simulink model "AircraftModel_6DoF_SAS"  (R2020b)
settings: Solver=VariableStepAuto  StartTime=0.0  StopTime=20  FixedStep=CNT_StepSize  RelTol=1e-3
values from neighbouring files (symbols this model uses):
  Actuators =     [ControlLaws.mat]    (also in MyTrimReport.mat; TrimState_1_LinearLatModel.mat; TrimState_1_LinearLatModel_Chi.mat; TrimState_1_LinearLatModel_Phasor.mat)
  Aerodynamics =     [ControlLaws.mat]    (also in MyTrimReport.mat; TrimState_1_LinearLatModel.mat; TrimState_1_LinearLatModel_Chi.mat; TrimState_1_LinearLatModel_Phasor.mat)
  CNT_a = 6378137    [AircraftParameters.m]    (also in ControlLaws.mat; MyTrimReport.mat; TrimState_1_LinearLatModel.mat; TrimState_1_LinearLatModel_Chi.mat)
  CNT_f = 0.003352810664747    (= 0.00335281066475)    [AircraftParameters.m]    (also in ControlLaws.mat; MyTrimReport.mat; TrimState_1_LinearLatModel.mat; TrimState_1_LinearLatModel_Chi.mat)
  CNT_g = [0;0;9.81]    [AircraftParameters.m]    (also in ControlLaws.mat = [0 0 9.81]; MyTrimReport.mat = [0 0 9.81]; TrimState_1_LinearLatModel.mat = [0 0 9.81]; TrimState_1_LinearLatModel_Chi.mat = [0 0 9.81])
  CNT_m = 15917    [AircraftParameters.m]    (also in ControlLaws.mat; MyTrimReport.mat; TrimState_1_LinearLatModel.mat; TrimState_1_LinearLatModel_Chi.mat)
  ControlLaws =     [ControlLaws.mat]    (also in MyTrimReport.mat; TrimState_1_LinearLatModel.mat; TrimState_1_LinearLatModel_Chi.mat; TrimState_1_LinearLatModel_Phasor.mat)
  Ixx = 105390    [AircraftParameters.m]    (also in ControlLaws.mat; MyTrimReport.mat; TrimState_1_LinearLatModel.mat; TrimState_1_LinearLatModel_Chi.mat)
  Ixz = 15539    [AircraftParameters.m]    (also in ControlLaws.mat; MyTrimReport.mat; TrimState_1_LinearLatModel.mat; TrimState_1_LinearLatModel_Chi.mat)
  Iyy = 280790    [AircraftParameters.m]    (also in ControlLaws.mat; MyTrimReport.mat; TrimState_1_LinearLatModel.mat; TrimState_1_LinearLatModel_Chi.mat)
  Izz = 350200    [AircraftParameters.m]    (also in ControlLaws.mat; MyTrimReport.mat; TrimState_1_LinearLatModel.mat; TrimState_1_LinearLatModel_Chi.mat)
  Propulsion =     [ControlLaws.mat]    (also in MyTrimReport.mat; TrimState_1_LinearLatModel.mat; TrimState_1_LinearLatModel_Chi.mat; TrimState_1_LinearLatModel_Phasor.mat)
  TrimPoint =     [ControlLaws.mat]    (also in MyTrimReport.mat; TrimState_1_LinearLatModel.mat; TrimState_1_LinearLatModel_Chi.mat; TrimState_1_LinearLatModel_Phasor.mat)
undefined symbols (not defined in the file or in its folder): ampl_p_cmd, beta_cmd, omega_p_cmd, TestSequence
libraries: simulink x32, vrlib x4
(part 1 of 2)
settings Model: Creator=NicolasS  LastModifiedBy=vlsag

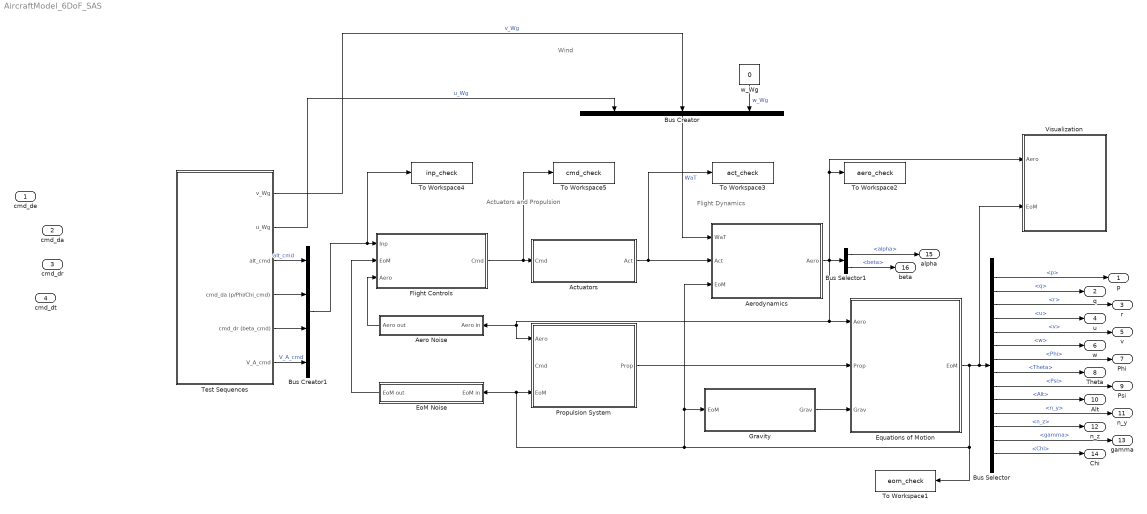
== system AircraftModel_6DoF_SAS ==
  note: Wind
  note: Actuators and Propulsion
  note: Flight Dynamics
  cmd_de : Inport
  cmd_da : Inport  Port=2
  cmd_dr : Inport  Port=3
  cmd_dt : Inport  Port=4
  Actuators : Subsystem
  Aero Noise : Subsystem
  Aerodynamics : Subsystem
  Bus Creator : BusCreator  Inputs=3
  Bus Creator1 : BusCreator  Inputs=4
  Bus Selector : BusSelector  OutputSignals=OOmega_f.p,OOmega_f.q,OOmega_f.r,vv_f.u,vv_f.v,vv_f.w,PPhi.Phi,PPhi.Theta,PPhi.Psi,Position.Alt,nn_f.n_y,nn_f.n_z,TrackData.gamma,TrackData.Chi
  Bus Selector1 : BusSelector  OutputSignals=AirData.alpha,AirData.beta
  EoM Noise : Subsystem
  Equations of Motion : Subsystem
  Flight Controls : Subsystem
  Gravity : Subsystem
  "Propulsion System " : Subsystem
  Test Sequences : Subsystem  InitFcn=|  StopFcn="clear beta_cmd  ampl_p_cmd omega_p_cmd tstart_p_cmd tstart_p_cmd TurnCompensation"
      | if not(exist('TestSequence','var'))
      | TestSequence = 7;
      | end
      | 
      | if not(exist('beta_cmd','var'))
      | beta_cmd = 0;
      | end
      | 
      | if not(exist('ampl_p_cmd','var'))
      | ampl_p_cmd = 0;
      | end
      | 
      | if not(exist('omega_p_cmd','var'))
      | omega_p_cmd = 0;
      | end
      | 
      | if not(exist('tstart_p_cmd','var'))
      | tstart_p_cmd = 0;
      | end
      | 
      | if not(exist('TurnCompensation','var'))
      |  if TestSequence == 4
      |     TurnCompensation = 0;
      |  else
      |     TurnCompensation = 1;
      |  end
      | end
  To Workspace1 : ToWorkspace  VariableName=eom_check  SaveFormat=Timeseries  SampleTime=-1
      settings: Decimation=2
  To Workspace2 : ToWorkspace  VariableName=aero_check  SaveFormat=Timeseries  SampleTime=-1
      settings: Decimation=2
  To Workspace3 : ToWorkspace  VariableName=act_check  SaveFormat=Timeseries  SampleTime=-1
      settings: Decimation=2
  To Workspace4 : ToWorkspace  VariableName=inp_check  SaveFormat=Timeseries  SampleTime=-1
      settings: Decimation=2
  To Workspace5 : ToWorkspace  VariableName=cmd_check  SaveFormat=Timeseries  SampleTime=-1
      settings: Decimation=2
  Visualization : Subsystem
  w_Wg : Constant  Value=0  SampleTime=-1
  p : Outport  Unit=rad/s
  q : Outport  Port=2  Unit=rad/s
  r : Outport  Port=3  Unit=rad/s
  u : Outport  Port=4  Unit=m/s
  v : Outport  Port=5  Unit=m/s
  w : Outport  Port=6  Unit=m/s
  Phi : Outport  Port=7  Unit=rad
  Theta : Outport  Port=8  Unit=rad
  Psi : Outport  Port=9  Unit=rad
  Alt : Outport  Port=10  Unit=m
  n_y : Outport  Port=11
  n_z : Outport  Port=12
  gamma : Outport  Port=13  Unit=rad
  Chi : Outport  Port=14  Unit=rad
  alpha : Outport  Port=15
  beta : Outport  Port=16
  wires:
  Test Sequences/2(u_Wg) -> Bus Creator/1  "u_Wg"
  Actuators/1(Act) -> To Workspace3/1, Aerodynamics/2(Act)
  Aerodynamics/1(Aero) -> To Workspace2/1, Visualization/1(Aero), Bus Selector1/1, Equations of Motion/1(Aero), Aero Noise/1(Aero in), "Propulsion System "/1(Aero)
  w_Wg/1 -> Bus Creator/3  "w_Wg"
  Equations of Motion/1(EoM) -> To Workspace1/1, Aerodynamics/3(EoM), Gravity/1(EoM), EoM Noise/1(EoM in), "Propulsion System "/3(EoM), Visualization/2(EoM), Bus Selector/1
  "Propulsion System "/1(Prop) -> Equations of Motion/2(Prop)
  Gravity/1(Grav) -> Equations of Motion/3(Grav)
  Bus Creator/1 -> Aerodynamics/1(WaT)  "WaT"
  Bus Selector1/2 -> beta/1  "<beta>"
  Test Sequences/1(v_Wg) -> Bus Creator/2  "v_Wg"
  Bus Selector/3 -> r/1  "<r>"
  Bus Selector/9 -> Psi/1  "<Psi>"
  Bus Selector/7 -> Phi/1  "<Phi>"
  Bus Selector/1 -> p/1  "<p>"
  Bus Selector/11 -> n_y/1  "<n_y>"
  Bus Selector1/1 -> alpha/1  "<alpha>"
  Bus Selector/2 -> q/1  "<q>"
  Bus Selector/6 -> w/1  "<w>"
  Bus Selector/4 -> u/1  "<u>"
  Bus Selector/12 -> n_z/1  "<n_z>"
  Bus Selector/10 -> Alt/1  "<Alt>"
  Bus Selector/8 -> Theta/1  "<Theta>"
  Bus Selector/13 -> gamma/1  "<gamma>"
  Bus Selector/14 -> Chi/1  "<Chi>"
  Bus Selector/5 -> v/1  "<v>"
  Flight Controls/1(Cmd) -> To Workspace5/1, Actuators/1(Cmd)
  Aero Noise/1(Aero out) -> Flight Controls/3(Aero)
  EoM Noise/1(EoM out) -> Flight Controls/2(EoM)
  Bus Creator1/1 -> To Workspace4/1, Flight Controls/1(Inp)
  Test Sequences/4(cmd_da (p/Phi/Chi_cmd)) -> Bus Creator1/2
  Test Sequences/3(alt_cmd) -> Bus Creator1/1  "alt_cmd"
  Test Sequences/5(cmd_dr (beta_cmd)) -> Bus Creator1/3
  Test Sequences/6(V_A_cmd) -> Bus Creator1/4  "V_A_cmd"

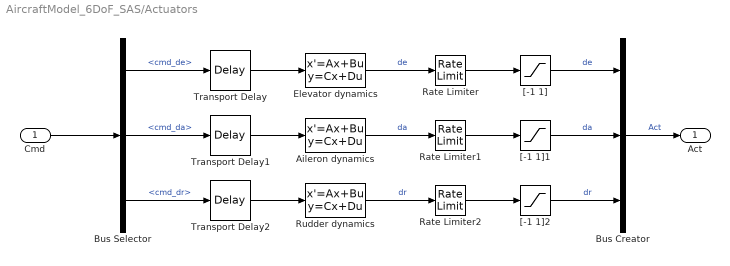
== system AircraftModel_6DoF_SAS/Actuators ==
  Cmd : Inport  OutDataTypeStr=Bus: Cmd
  Aileron dynamics : StateSpace  A=Actuators.Act_a.A  B=Actuators.Act_a.B  C=Actuators.Act_a.C  D=Actuators.Act_a.D  InitialCondition=TrimPoint.States.dabar  ContinuousStateAttributes='da'
  Bus Creator : BusCreator  Inputs=3  OutDataTypeStr=Bus: Act
  Bus Selector : BusSelector  OutputSignals=cmd_de,cmd_da,cmd_dr
  Elevator dynamics : StateSpace  A=Actuators.Act_e.A  B=Actuators.Act_e.B  C=Actuators.Act_e.C  D=Actuators.Act_e.D  InitialCondition=TrimPoint.States.debar  ContinuousStateAttributes='de'
  Rate Limiter : RateLimiter  RisingSlewLimit=max(Actuators.RateLimits.udot_max_He)  FallingSlewLimit=min(Actuators.RateLimits.udot_max_He)  SampleTimeMode=inherited
  Rate Limiter1 : RateLimiter  RisingSlewLimit=max(Actuators.RateLimits.udot_max_Ha)  FallingSlewLimit=min(Actuators.RateLimits.udot_max_Ha)  SampleTimeMode=inherited
  Rate Limiter2 : RateLimiter  RisingSlewLimit=max(Actuators.RateLimits.udot_max_Hr)  FallingSlewLimit=min(Actuators.RateLimits.udot_max_Hr)  SampleTimeMode=inherited
  Rudder dynamics : StateSpace  A=Actuators.Act_r.A  B=Actuators.Act_r.B  C=Actuators.Act_r.C  D=Actuators.Act_r.D  InitialCondition=TrimPoint.States.drbar  ContinuousStateAttributes='dr'
  Transport Delay : TransportDelay  DelayTime=Actuators.Delays.tau_de  InitialOutput=TrimPoint.States.debar  TransDelayFeedthrough=on
  Transport Delay1 : TransportDelay  DelayTime=Actuators.Delays.tau_da  InitialOutput=TrimPoint.States.dabar  TransDelayFeedthrough=on
  Transport Delay2 : TransportDelay  DelayTime=Actuators.Delays.tau_dr  InitialOutput=TrimPoint.States.drbar  TransDelayFeedthrough=on
  "[-1 1]" : Saturate  UpperLimit=max(Actuators.Limits.u_max_He)  LowerLimit=min(Actuators.Limits.u_max_He)
  "[-1 1]1" : Saturate  UpperLimit=max(Actuators.Limits.u_max_Ha)  LowerLimit=min(Actuators.Limits.u_max_Ha)
  "[-1 1]2" : Saturate  UpperLimit=max(Actuators.Limits.u_max_Hr)  LowerLimit=min(Actuators.Limits.u_max_Hr)
  Act : Outport  OutDataTypeStr=Bus: Act
  wires:
  Elevator dynamics/1 -> Rate Limiter/1  "de"
  "[-1 1]1"/1 -> Bus Creator/2  "da"
  Rudder dynamics/1 -> Rate Limiter2/1  "dr"
  Transport Delay1/1 -> Aileron dynamics/1
  Cmd/1 -> Bus Selector/1
  "[-1 1]"/1 -> Bus Creator/1  "de"
  Bus Selector/1 -> Transport Delay/1  "<cmd_de>"
  Transport Delay/1 -> Elevator dynamics/1
  "[-1 1]2"/1 -> Bus Creator/3  "dr"
  Transport Delay2/1 -> Rudder dynamics/1
  Aileron dynamics/1 -> Rate Limiter1/1  "da"
  Bus Selector/3 -> Transport Delay2/1  "<cmd_dr>"
  Bus Creator/1 -> Act/1  "Act"
  Bus Selector/2 -> Transport Delay1/1  "<cmd_da>"
  Rate Limiter/1 -> "[-1 1]"/1
  Rate Limiter1/1 -> "[-1 1]1"/1
  Rate Limiter2/1 -> "[-1 1]2"/1

== system AircraftModel_6DoF_SAS/Aero Noise ==
  Aero in : Inport  OutDataTypeStr=Bus: Aero
  Band-Limited White Noise1 : simulink/Sources/Band-Limited White Noise  Cov=1E-7  Ts=0.01  seed=5749
  Band-Limited White Noise8 : simulink/Sources/Band-Limited White Noise  Cov=1E-7  Ts=0.01  seed=3324
  Band-Limited White Noise9 : simulink/Sources/Band-Limited White Noise  Cov=1E-3  Ts=0.05  seed=8153
  Bus Creator2 : BusCreator  Inputs=7  OutDataTypeStr=Bus: Aero
  Bus Creator3 : BusCreator  Inputs=7  OutDataTypeStr=Bus: AirData
  Bus Selector : BusSelector  OutputSignals=AirData.u_Af,AirData.v_Af,AirData.w_Af,AirData.V_A,AirData.p_dyn,AirData.alpha,AirData.beta,X_A,Y_A,Z_A,L_A,M_A,N_A
  Sum1 : Sum  Inputs=++|
  Sum2 : Sum  Inputs=++|
  Sum3 : Sum  Inputs=++|
  Aero out : Outport  OutDataTypeStr=Bus: Aero
  wires:
  Aero in/1 -> Bus Selector/1
  Bus Creator3/1 -> Bus Creator2/1  "AirData"
  Bus Selector/7 -> Sum2/2  "<beta>"
  Bus Selector/8 -> Bus Creator2/2  "<X_A>"
  Bus Creator2/1 -> Aero out/1  "Aero"
  Bus Selector/1 -> Bus Creator3/1  "<u_Af>"
  Bus Selector/3 -> Bus Creator3/3  "<w_Af>"
  Bus Selector/4 -> Sum3/2  "<V_A>"
  Bus Selector/6 -> Sum1/2  "<alpha>"
  Band-Limited White Noise8/1 -> Sum1/1
  Sum1/1 -> Bus Creator3/6  "alpha"
  Bus Selector/5 -> Bus Creator3/5  "<p_dyn>"
  Band-Limited White Noise9/1 -> Sum3/1
  Sum3/1 -> Bus Creator3/4  "V_A"
  Bus Selector/2 -> Bus Creator3/2  "<v_Af>"
  Bus Selector/9 -> Bus Creator2/3  "<Y_A>"
  Bus Selector/10 -> Bus Creator2/4  "<Z_A>"
  Bus Selector/11 -> Bus Creator2/5  "<L_A>"
  Bus Selector/12 -> Bus Creator2/6  "<M_A>"
  Bus Selector/13 -> Bus Creator2/7  "<N_A>"
  Band-Limited White Noise1/1 -> Sum2/1
  Sum2/1 -> Bus Creator3/7  "beta"

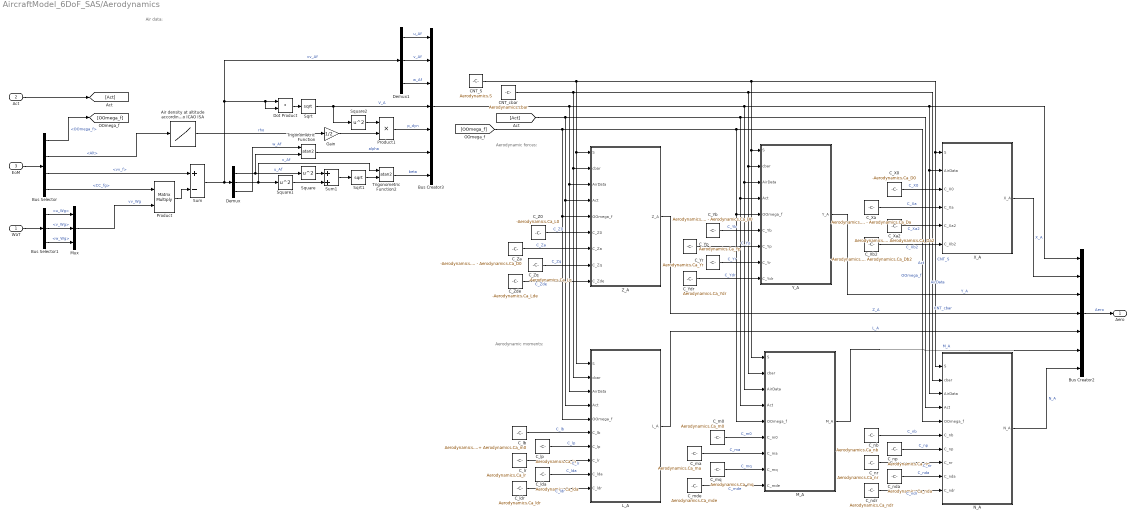
== system AircraftModel_6DoF_SAS/Aerodynamics ==
  note: Air data:
  note: Aerodynamic moments:
  note: Aerodynamic forces:
  WaT : Inport  OutDataTypeStr=Bus: WaT
  Act : Inport  Port=2  OutDataTypeStr=Bus: Act
  EoM : Inport  Port=3  OutDataTypeStr=Bus: EoM
  Air density at altitude according to ICAO ISA : Lookup_n-D  NumberOfTableDimensions=1  BreakpointsForDimension1=Aerodynamics.LUT_Alt  Table=Aerodynamics.LUT_rho  ExtrapMethod=Clip  InternalRulePriority=Speed  RndMeth=Simplest  InputSameDT=on
  Bus Creator2 : BusCreator  Inputs=7  OutDataTypeStr=Bus: Aero
  Bus Creator3 : BusCreator  Inputs=7  OutDataTypeStr=Bus: AirData
  Bus Selector : BusSelector  OutputSignals=OOmega_f,Position.Alt,vv_f,CC.CC_fg
  Bus Selector1 : BusSelector  OutputSignals=u_Wg,v_Wg,w_Wg
  CNT_S : Constant  Value=Aerodynamics.S  OutDataTypeStr=double  SampleTime=-1
  CNT_cbar : Constant  Value=Aerodynamics.cbar  OutDataTypeStr=double  SampleTime=-1
  C_X0 : Constant  Value=-Aerodynamics.Ca_D0  VectorParams1D=off  OutDataTypeStr=double  SampleTime=-1
  C_Xa : Constant  Value=Aerodynamics.Ca_L0 - Aerodynamics.Ca_Da  VectorParams1D=off  OutDataTypeStr=double  SampleTime=-1
  C_Xa2 : Constant  Value=Aerodynamics.Ca_La - Aerodynamics.Ca_Da2  VectorParams1D=off  OutDataTypeStr=double  SampleTime=-1
  C_Xb2 : Constant  Value=-Aerodynamics.Ca_Yb - Aerodynamics.Ca_Db2  VectorParams1D=off  OutDataTypeStr=double  SampleTime=-1
  C_Yb : Constant  Value=Aerodynamics.Ca_Yb - Aerodynamics.Ca_D0  VectorParams1D=off  OutDataTypeStr=double  SampleTime=-1
  C_Ydr : Constant  Value=Aerodynamics.Ca_Ydr  VectorParams1D=off  OutDataTypeStr=double  SampleTime=-1
  C_Yp : Constant  Value=Aerodynamics.Ca_Yp  VectorParams1D=off  OutDataTypeStr=double  SampleTime=-1
  C_Yr : Constant  Value=Aerodynamics.Ca_Yr  VectorParams1D=off  OutDataTypeStr=double  SampleTime=-1
  C_Z0 : Constant  Value=-Aerodynamics.Ca_L0  VectorParams1D=off  OutDataTypeStr=double  SampleTime=-1
  C_Za : Constant  Value=-Aerodynamics.Ca_La - Aerodynamics.Ca_D0  VectorParams1D=off  OutDataTypeStr=double  SampleTime=-1
  C_Zde : Constant  Value=-Aerodynamics.Ca_Lde  VectorParams1D=off  OutDataTypeStr=double  SampleTime=-1
  C_Zq : Constant  Value=-Aerodynamics.Ca_Lq  VectorParams1D=off  OutDataTypeStr=double  SampleTime=-1
  C_lb : Constant  Value=Aerodynamics.Ca_lb + Aerodynamics.Ca_m0  VectorParams1D=off  OutDataTypeStr=double  SampleTime=-1
  C_lda : Constant  Value=Aerodynamics.Ca_lda  VectorParams1D=off  OutDataTypeStr=double  SampleTime=-1
  C_ldr : Constant  Value=Aerodynamics.Ca_ldr  VectorParams1D=off  OutDataTypeStr=double  SampleTime=-1
  C_lp : Constant  Value=Aerodynamics.Ca_lp  VectorParams1D=off  OutDataTypeStr=double  SampleTime=-1
  C_lr : Constant  Value=Aerodynamics.Ca_lr  VectorParams1D=off  OutDataTypeStr=double  SampleTime=-1
  C_m0 : Constant  Value=Aerodynamics.Ca_m0  VectorParams1D=off  OutDataTypeStr=double  SampleTime=-1
  C_ma : Constant  Value=Aerodynamics.Ca_ma  VectorParams1D=off  OutDataTypeStr=double  SampleTime=-1
  C_mde : Constant  Value=Aerodynamics.Ca_mde  VectorParams1D=off  OutDataTypeStr=double  SampleTime=-1
  C_mq : Constant  Value=Aerodynamics.Ca_mq  VectorParams1D=off  OutDataTypeStr=double  SampleTime=-1
  C_nb : Constant  Value=Aerodynamics.Ca_nb  VectorParams1D=off  OutDataTypeStr=double  SampleTime=-1
  C_nda : Constant  Value=Aerodynamics.Ca_nda  VectorParams1D=off  OutDataTypeStr=double  SampleTime=-1
  C_ndr : Constant  Value=Aerodynamics.Ca_ndr  VectorParams1D=off  OutDataTypeStr=double  SampleTime=-1
  C_np : Constant  Value=Aerodynamics.Ca_np  VectorParams1D=off  OutDataTypeStr=double  SampleTime=-1
  C_nr : Constant  Value=Aerodynamics.Ca_nr  VectorParams1D=off  OutDataTypeStr=double  SampleTime=-1
  Demux : Demux  Outputs=3
  Demux1 : Demux  Outputs=3
  Dot Product : DotProduct  InputSameDT=on  OutDataTypeStr=Inherit: Inherit via internal rule
  Gain : Gain  Gain=1/2
  L_A : MATLAB Function  TreatAsAtomicUnit=on
  M_A : MATLAB Function  TreatAsAtomicUnit=on
  Mux : Mux  Inputs=3
  N_A : MATLAB Function  TreatAsAtomicUnit=on
  Product : Product  Multiplication=Matrix(*)
  Product1 : Product
  Sqrt : Sqrt  SaturateOnIntegerOverflow=on
  Sqrt1 : Sqrt  SaturateOnIntegerOverflow=on
  Square : Math  Operator=square  SaturateOnIntegerOverflow=on
  Square1 : Math  Operator=square  SaturateOnIntegerOverflow=on
  Square2 : Math  Operator=square  SaturateOnIntegerOverflow=on
  Sum : Sum  Inputs=+-
  Sum1 : Sum
  Trigonometric Function : Trigonometry  Operator=atan2
  Trigonometric Function2 : Trigonometry  Operator=atan2
  X_A : MATLAB Function  TreatAsAtomicUnit=on
  Y_A : MATLAB Function  TreatAsAtomicUnit=on
  Z_A : MATLAB Function  TreatAsAtomicUnit=on
  Aero : Outport  OutDataTypeStr=Bus: Aero
  wires:
  Demux1/3 -> Bus Creator3/3  "w_Af"
  C_lp/1 -> L_A/7(C_lp)  "C_lp"
  Act/1 -> [Act]
  N_A/1(N_A) -> Bus Creator2/7  "N_A"
  C_nb/1 -> N_A/6(C_nb)  "C_nb"
  C_ldr/1 -> L_A/10(C_ldr)  "C_ldr"
  C_m0/1 -> M_A/6(C_m0)  "C_m0"
  C_Zq/1 -> Z_A/8(C_Zq)  "C_Zq"
  [OOmega_f] -> N_A/5(OOmega_f), M_A/5(OOmega_f), Y_A/5(OOmega_f), L_A/5(OOmega_f), Z_A/5(OOmega_f)  "OOmega_f"
  C_lr/1 -> L_A/8(C_lr)  "C_lr"
  C_mq/1 -> M_A/8(C_mq)  "C_mq"
  Air density at altitude according to ICAO ISA/1 -> Gain/1  "rho"
  C_Z0/1 -> Z_A/6(C_Z0)  "C_Z0"
  Square/1 -> Sum1/1
  X_A/1(X_A) -> Bus Creator2/2  "X_A"
  Trigonometric Function2/1 -> Bus Creator3/7  "beta"
  C_Yr/1 -> Y_A/8(C_Yr)  "C_Yr"
  C_Yb/1 -> Y_A/6(C_Yb)  "C_Yb"
  Demux1/2 -> Bus Creator3/2  "v_Af"
  Dot Product/1 -> Sqrt/1
  C_ma/1 -> M_A/7(C_ma)  "C_ma"
  C_nda/1 -> N_A/9(C_nda)  "C_nda"
  C_Xa/1 -> X_A/4(C_Xa)  "C_Xa"
  C_lb/1 -> L_A/6(C_lb)  "C_lb"
  Sum/1 -> Demux/1, Demux1/1, Dot Product/2, Dot Product/1  "vv_Af"
  C_Xa2/1 -> X_A/5(C_Xa2)  "C_Xa2"
  C_Ydr/1 -> Y_A/9(C_Ydr)  "C_Ydr"
  C_Xb2/1 -> X_A/6(C_Xb2)  "C_Xb2"
  Y_A/1(Y_A) -> Bus Creator2/3  "Y_A"
  C_Za/1 -> Z_A/7(C_Za)  "C_Za"
  CNT_S/1 -> N_A/1(S), X_A/1(S), M_A/1(S), Y_A/1(S), L_A/1(S), Z_A/1(S)  "CNT_S"
  C_nr/1 -> N_A/8(C_nr)  "C_nr"
  Bus Creator2/1 -> Aero/1  "Aero"
  C_mde/1 -> M_A/9(C_mde)  "C_mde"
  [Act] -> N_A/4(Act), M_A/4(Act), Y_A/4(Act), L_A/4(Act), Z_A/4(Act)  "Act"
  Demux/3 -> Trigonometric Function/1  "w_Af"
  C_X0/1 -> X_A/3(C_X0)  "C_X0"
  C_np/1 -> N_A/7(C_np)  "C_np"
  Demux/2 -> Square1/1, Trigonometric Function2/1  "v_Af"
  C_Yp/1 -> Y_A/7(C_Yp)  "C_Yp"
  C_ndr/1 -> N_A/10(C_ndr)  "C_ndr"
  Demux/1 -> Square/1, Trigonometric Function/2  "u_Af"
  Bus Creator3/1 -> L_A/3(AirData), Z_A/3(AirData), Bus Creator2/1, N_A/3(AirData), X_A/2(AirData), M_A/3(AirData), Y_A/3(AirData)  "AirData"
  M_A/1(M_A) -> Bus Creator2/6  "M_A"
  Sqrt1/1 -> Trigonometric Function2/2
  Bus Selector/2 -> Air density at altitude according to ICAO ISA/1  "<Alt>"
  C_Zde/1 -> Z_A/9(C_Zde)  "C_Zde"
  Gain/1 -> Product1/2
  Product/1 -> Sum/2
  C_lda/1 -> L_A/9(C_lda)  "C_lda"
  L_A/1(L_A) -> Bus Creator2/5  "L_A"
  Demux1/1 -> Bus Creator3/1  "u_Af"
  Z_A/1(Z_A) -> Bus Creator2/4  "Z_A"
  Product1/1 -> Bus Creator3/5  "p_dyn"
  Sqrt/1 -> Square2/1, Bus Creator3/4  "V_A"
  CNT_cbar/1 -> N_A/2(cbar), M_A/2(cbar), Y_A/2(cbar), L_A/2(cbar), Z_A/2(cbar)  "CNT_cbar"
  Trigonometric Function/1 -> Bus Creator3/6  "alpha"
  Bus Selector/3 -> Sum/1  "<vv_f>"
  Sum1/1 -> Sqrt1/1
  EoM/1 -> Bus Selector/1
  Bus Selector/1 -> [OOmega_f]  "<OOmega_f>"
  Bus Selector/4 -> Product/1  "<CC_fg>"
  Square2/1 -> Product1/1
  Square1/1 -> Sum1/2
  WaT/1 -> Bus Selector1/1
  Bus Selector1/1 -> Mux/1  "<u_Wg>"
  Bus Selector1/2 -> Mux/2  "<v_Wg>"
  Bus Selector1/3 -> Mux/3  "<w_Wg>"
  Mux/1 -> Product/2  "vv_Wg"

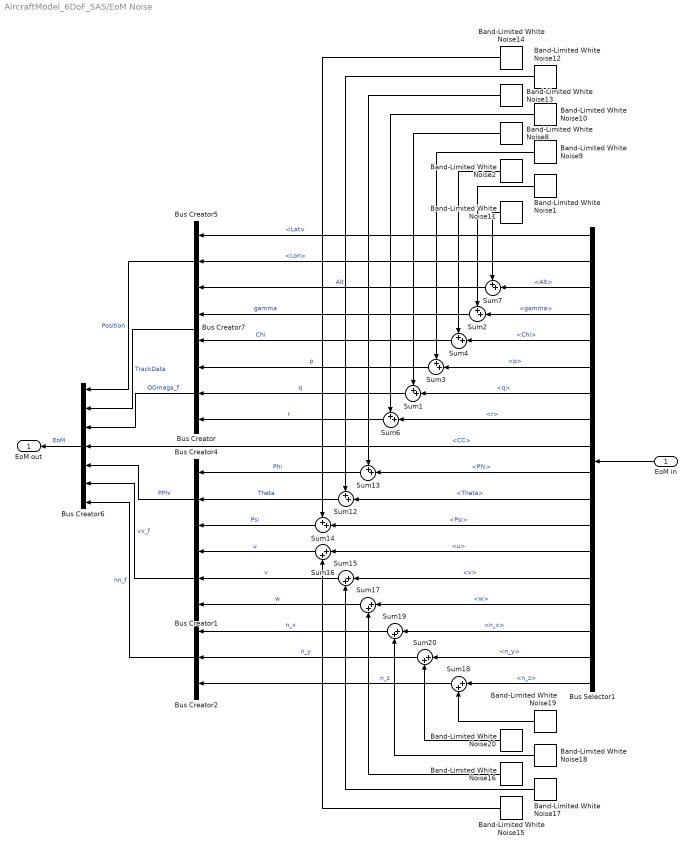
== system AircraftModel_6DoF_SAS/EoM Noise ==
  EoM in : Inport  OutDataTypeStr=Bus: EoM
  Band-Limited White Noise1 : simulink/Sources/Band-Limited White Noise  Cov=1E-7  Ts=0.01  seed=1102
  Band-Limited White Noise10 : simulink/Sources/Band-Limited White Noise  Cov=1E-6  Ts=0.01  seed=66897
  Band-Limited White Noise11 : simulink/Sources/Band-Limited White Noise  Cov=1E-4  Ts=0.1  seed=6874
  Band-Limited White Noise12 : simulink/Sources/Band-Limited White Noise  Cov=5E-7  Ts=0.01  seed=45875
  Band-Limited White Noise13 : simulink/Sources/Band-Limited White Noise  Cov=5E-7  Ts=0.01  seed=74148
  Band-Limited White Noise14 : simulink/Sources/Band-Limited White Noise  Cov=5E-7  Ts=0.01  seed=3514
  Band-Limited White Noise15 : simulink/Sources/Band-Limited White Noise  Cov=5E-5  Ts=0.1  seed=54769
  Band-Limited White Noise16 : simulink/Sources/Band-Limited White Noise  Cov=1E-4  Ts=0.01  seed=6932
  Band-Limited White Noise17 : simulink/Sources/Band-Limited White Noise  Cov=1E-4  Ts=0.01  seed=4485
  Band-Limited White Noise18 : simulink/Sources/Band-Limited White Noise  Cov=1E-5  Ts=0.01  seed=11452
  Band-Limited White Noise19 : simulink/Sources/Band-Limited White Noise  Cov=1E-5  Ts=0.01  seed=3324
  Band-Limited White Noise2 : simulink/Sources/Band-Limited White Noise  Cov=1E-7  Ts=0.1  seed=2201
  Band-Limited White Noise20 : simulink/Sources/Band-Limited White Noise  Cov=1E-5  Ts=0.01  seed=58967
  Band-Limited White Noise8 : simulink/Sources/Band-Limited White Noise  Cov=1E-6  Ts=0.01  seed=[23341]
  Band-Limited White Noise9 : simulink/Sources/Band-Limited White Noise  Cov=1E-6  Ts=0.01  seed=1147
  Bus Creator : BusCreator  Inputs=3  OutDataTypeStr=Bus: OOmega_f
  Bus Creator1 : BusCreator  Inputs=3  OutDataTypeStr=Bus: vv_f
  Bus Creator2 : BusCreator  Inputs=3  OutDataTypeStr=Bus: nn_f
  Bus Creator4 : BusCreator  Inputs=3  OutDataTypeStr=Bus: PPhi
  Bus Creator5 : BusCreator  Inputs=3  OutDataTypeStr=Bus: Position
  Bus Creator6 : BusCreator  Inputs=7  OutDataTypeStr=Bus: EoM
  Bus Creator7 : BusCreator  Inputs=2  OutDataTypeStr=Bus: TrackData
  Bus Selector1 : BusSelector  OutputSignals=Position.Lat,Position.Lon,Position.Alt,TrackData.gamma,TrackData.Chi,OOmega_f.p,OOmega_f.q,OOmega_f.r,CC,PPhi.Phi,PPhi.Theta,PPhi.Psi,vv_f.u,vv_f.v,vv_f.w,nn_f.n_x,nn_f.n_y,nn_f.n_z
  Sum{1..4,6..7,12..14} (9 alike) : Sum  Inputs=++|
  Sum{15..20} (6 alike) : Sum  Inputs=|++
  EoM out : Outport  OutDataTypeStr=Bus: EoM
  wires:
  EoM in/1 -> Bus Selector1/1
  Bus Selector1/6 -> Sum3/2  "<p>"
  Bus Selector1/7 -> Sum1/2  "<q>"
  Band-Limited White Noise9/1 -> Sum3/1
  Bus Selector1/8 -> Sum6/2  "<r>"
  Band-Limited White Noise10/1 -> Sum6/1
  Band-Limited White Noise11/1 -> Sum7/1
  Bus Selector1/3 -> Sum7/2  "<Alt>"
  Band-Limited White Noise12/1 -> Sum12/1
  Bus Selector1/10 -> Sum13/2  "<Phi>"
  Bus Selector1/11 -> Sum12/2  "<Theta>"
  Bus Selector1/12 -> Sum14/2  "<Psi>"
  Band-Limited White Noise13/1 -> Sum13/1
  Band-Limited White Noise14/1 -> Sum14/1
  Bus Selector1/16 -> Sum19/1  "<n_x>"
  Bus Selector1/17 -> Sum20/1  "<n_y>"
  Bus Selector1/18 -> Sum18/1  "<n_z>"
  Bus Selector1/15 -> Sum17/1  "<w>"
  Bus Selector1/13 -> Sum16/1  "<u>"
  Band-Limited White Noise16/1 -> Sum17/2
  Band-Limited White Noise15/1 -> Sum16/2
  Bus Selector1/14 -> Sum15/1  "<v>"
  Band-Limited White Noise17/1 -> Sum15/2
  Band-Limited White Noise19/1 -> Sum18/2
  Band-Limited White Noise18/1 -> Sum19/2
  Band-Limited White Noise20/1 -> Sum20/2
  Bus Selector1/1 -> Bus Creator5/1  "<Lat>"
  Bus Selector1/2 -> Bus Creator5/2  "<Lon>"
  Sum19/1 -> Bus Creator2/1  "n_x"
  Sum20/1 -> Bus Creator2/2  "n_y"
  Sum18/1 -> Bus Creator2/3  "n_z"
  Sum15/1 -> Bus Creator1/2  "v"
  Sum16/1 -> Bus Creator1/1  "u"
  Sum17/1 -> Bus Creator1/3  "w"
  Sum7/1 -> Bus Creator5/3  "Alt"
  Sum6/1 -> Bus Creator/3  "r"
  Sum1/1 -> Bus Creator/2  "q"
  Sum3/1 -> Bus Creator/1  "p"
  Sum13/1 -> Bus Creator4/1  "Phi"
  Bus Selector1/9 -> Bus Creator6/4  "<CC>"
  Sum12/1 -> Bus Creator4/2  "Theta"
  Sum14/1 -> Bus Creator4/3  "Psi"
  Bus Creator5/1 -> Bus Creator6/1  "Position"
  Bus Creator/1 -> Bus Creator6/3  "OOmega_f"
  Bus Creator4/1 -> Bus Creator6/5  "PPhi"
  Bus Creator1/1 -> Bus Creator6/6  "vv_f"
  Bus Creator2/1 -> Bus Creator6/7  "nn_f"
  Bus Creator6/1 -> EoM out/1  "EoM"
  Band-Limited White Noise8/1 -> Sum1/1
  Bus Creator7/1 -> Bus Creator6/2  "TrackData"
  Band-Limited White Noise1/1 -> Sum2/1
  Bus Selector1/5 -> Sum4/2  "<Chi>"
  Band-Limited White Noise2/1 -> Sum4/1
  Bus Selector1/4 -> Sum2/2  "<gamma>"
  Sum2/1 -> Bus Creator7/1  "gamma"
  Sum4/1 -> Bus Creator7/2  "Chi"

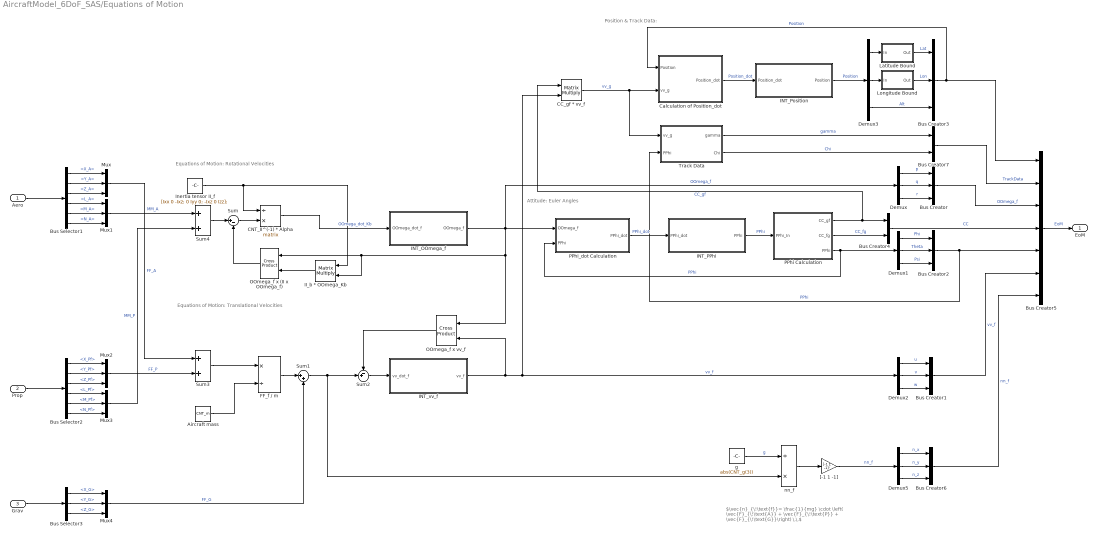
== system AircraftModel_6DoF_SAS/Equations of Motion ==
  note: Equations of Motion: Translational Velocities
  note: Equations of Motion: Rotational Velocities
  note: Attitude: Euler Angles
  note: Position & Track Data:
  note: $\vec{n}_{\!\text{f}}= \frac{1}{mg} \cdot \left( \vec{F}_{\!\text{A}} + \vec{F}_{\!\text{P}} + \vec{F}_{\!\text{G}}\right) \,\,$
  Aero : Inport  OutDataTypeStr=Bus: Aero
  Prop : Inport  Port=2  OutDataTypeStr=Bus: Prop
  Grav : Inport  Port=3  OutDataTypeStr=Bus: Grav
  Aircraft mass : Constant  Value=CNT_m  SampleTime=-1
  Bus Creator : BusCreator  Inputs=3  OutDataTypeStr=Bus: OOmega_f
  Bus Creator1 : BusCreator  Inputs=3  OutDataTypeStr=Bus: vv_f
  Bus Creator2 : BusCreator  Inputs=3  OutDataTypeStr=Bus: PPhi
  Bus Creator3 : BusCreator  Inputs=3  OutDataTypeStr=Bus: Position
  Bus Creator4 : BusCreator  Inputs=2  OutDataTypeStr=Bus: CC
  Bus Creator5 : BusCreator  Inputs=7  OutDataTypeStr=Bus: EoM
  Bus Creator6 : BusCreator  Inputs=3  OutDataTypeStr=Bus: nn_f
  Bus Creator7 : BusCreator  Inputs=2  OutDataTypeStr=Bus: TrackData
  Bus Selector1 : BusSelector  OutputSignals=X_A,Y_A,Z_A,L_A,M_A,N_A
  Bus Selector2 : BusSelector  OutputSignals=X_Pf,Y_Pf,Z_Pf,L_Pf,M_Pf,N_Pf
  Bus Selector3 : BusSelector  OutputSignals=X_G,Y_G,Z_G
  CC_gf * vv_f : Product  Multiplication=Matrix(*)  RndMeth=Zero
  CNT_II^(-1) * Alpha : Product  Inputs=/*  Multiplication=Matrix(*)
  Calculation of Position_dot : Subsystem
  Demux{,1..3,5} (5 alike) : Demux  Outputs=3
  FF_f / m : Product  Inputs=*/
  II_b * OOmega_Kb : Product  Multiplication=Matrix(*)  RndMeth=Zero
  INT_OOmega_f : Subsystem
  INT_PPhi : Subsystem
  INT_Position : Subsystem
  INT_vv_f : Subsystem
  Inertia tensor II_f : Constant  Value=[Ixx 0 -Ixz; 0 Iyy 0; -Ixz 0 Izz];  SampleTime=-1
  Latitude Bound : Subsystem  mask(Latitude bound){}
      mask help: Bounds the latitude to [-pi/2, pi/2]. When the lower bound is exceeded the latitude is increasing again; when the upper bound is exceeded the latitude is decreasing.
  Longitude Bound : Subsystem  mask(Longitude bound){}
      mask help: Bounds the longitude to [-pi, pi]. When -pi bound is exceeded the longitude wraps back to pi; when the pi bound is exceeded the longitude wraps back to -pi.
  Mux{,1..4} (5 alike) : Mux  Inputs=3
  OOmega_f x (II x OOmega_f) : vrlib/Utilities/Cross Product
  OOmega_f x vv_f : vrlib/Utilities/Cross Product
  PPhi Calculation : MATLAB Function  TreatAsAtomicUnit=on
  PPhi_dot Calculation : MATLAB Function  TreatAsAtomicUnit=on
  Sum : Sum  Inputs=|+-
  Sum1 : Sum  Inputs=|++
  Sum2 : Sum  Inputs=-+|
  Sum3 : Sum
  Sum4 : Sum
  Track Data : Subsystem
  "[-1 1 -1]" : Gain  Gain=[-1 1 -1]'
  g : Constant  Value=abs(CNT_g(3))  SampleTime=-1
  "nn_f " : Product  Inputs=/*  RndMeth=Zero
  EoM : Outport  OutDataTypeStr=Bus: EoM
  wires:
  Longitude Bound/1(Out) -> Bus Creator3/2  "Lon"
  "[-1 1 -1]"/1 -> Demux5/1  "nn_f"
  Bus Selector1/6 -> Mux1/3  "<N_A>"
  Bus Creator/1 -> Bus Creator5/3  "OOmega_f"
  Bus Selector2/5 -> Mux3/2  "<M_Pf>"
  INT_OOmega_f/1(OOmega_f) -> Demux/1, II_b * OOmega_Kb/2, OOmega_f x (II x OOmega_f)/1, OOmega_f x vv_f/1, PPhi_dot Calculation/1(OOmega_f)  "OOmega_f"
  Demux/2 -> Bus Creator/2  "q"
  Prop/1 -> Bus Selector2/1
  Mux1/1 -> Sum4/1  "MM_A"
  Demux/1 -> Bus Creator/1  "p"
  Demux1/2 -> Bus Creator2/2  "Theta"
  Bus Creator1/1 -> Bus Creator5/6  "vv_f"
  Demux3/2 -> Longitude Bound/1(In)
  INT_vv_f/1(vv_f) -> Demux2/1, CC_gf * vv_f/2, OOmega_f x vv_f/2  "vv_f"
  Mux2/1 -> Sum3/2  "FF_P"
  "nn_f "/1 -> "[-1 1 -1]"/1
  Demux2/3 -> Bus Creator1/3  "w"
  Bus Selector2/3 -> Mux2/3  "<Z_Pf>"
  Demux5/1 -> Bus Creator6/1  "n_x"
  Bus Creator6/1 -> Bus Creator5/7  "nn_f"
  Demux5/2 -> Bus Creator6/2  "n_y"
  Demux/3 -> Bus Creator/3  "r"
  OOmega_f x vv_f/1 -> Sum2/1
  Bus Selector2/2 -> Mux2/2  "<Y_Pf>"
  g/1 -> "nn_f "/1  "g"
  Bus Selector1/3 -> Mux/3  "<Z_A>"
  Mux/1 -> Sum3/1  "FF_A"
  PPhi Calculation/1(CC_gf) -> CC_gf * vv_f/1, Bus Creator4/1  "CC_gf"
  Bus Selector1/4 -> Mux1/1  "<L_A>"
  INT_PPhi/1(PPhi) -> PPhi Calculation/1(PPhi_In)  "PPhi"
  PPhi Calculation/3(PPhi) -> PPhi_dot Calculation/2(PPhi), Demux1/1  "PPhi"
  Bus Creator3/1 -> Bus Creator5/1, Calculation of Position_dot/1(Position)  "Position"
  CC_gf * vv_f/1 -> Track Data/1(vv_g), Calculation of Position_dot/2(vv_g)  "vv_g"
  Mux3/1 -> Sum4/2  "MM_P"
  Aircraft mass/1 -> FF_f / m/2
  PPhi Calculation/2(CC_fg) -> Bus Creator4/2  "CC_fg"
  Aero/1 -> Bus Selector1/1
  Calculation of Position_dot/1(Position_dot) -> INT_Position/1(Position_dot)  "Position_dot"
  Demux3/3 -> Bus Creator3/3  "Alt"
  Sum3/1 -> FF_f / m/1
  Bus Selector1/2 -> Mux/2  "<Y_A>"
  Demux2/1 -> Bus Creator1/1  "u"
  Sum2/1 -> INT_vv_f/1(vv_dot_f)
  Demux2/2 -> Bus Creator1/2  "v"
  PPhi_dot Calculation/1(PPhi_dot) -> INT_PPhi/1(PPhi_dot)  "PPhi_dot"
  Bus Creator2/1 -> Track Data/2(PPhi), Bus Creator5/5  "PPhi"
  Bus Creator4/1 -> Bus Creator5/4  "CC"
  OOmega_f x (II x OOmega_f)/1 -> Sum/2
  Latitude Bound/1(Out) -> Bus Creator3/1  "Lat"
  Sum1/1 -> "nn_f "/2, Sum2/2
  FF_f / m/1 -> Sum1/1
  II_b * OOmega_Kb/1 -> OOmega_f x (II x OOmega_f)/2
  Bus Selector1/5 -> Mux1/2  "<M_A>"
  Demux1/1 -> Bus Creator2/1  "Phi"
  Bus Selector2/1 -> Mux2/1  "<X_Pf>"
  Sum/1 -> CNT_II^(-1) * Alpha/2
  Demux3/1 -> Latitude Bound/1(In)
  Bus Selector2/4 -> Mux3/1  "<L_Pf>"
  Demux1/3 -> Bus Creator2/3  "Psi"
  INT_Position/1(Position) -> Demux3/1  "Position"
  Inertia tensor II_f/1 -> CNT_II^(-1) * Alpha/1, II_b * OOmega_Kb/1
  Bus Selector1/1 -> Mux/1  "<X_A>"
  CNT_II^(-1) * Alpha/1 -> INT_OOmega_f/1(OOmega_dot_f)  "OOmega_dot_Kb"
  Bus Selector2/6 -> Mux3/3  "<N_Pf>"
  Sum4/1 -> Sum/1
  Demux5/3 -> Bus Creator6/3  "n_z"
  Bus Creator5/1 -> EoM/1  "EoM"
  Mux4/1 -> Sum1/2  "FF_G"
  Bus Selector3/1 -> Mux4/1  "<X_G>"
  Grav/1 -> Bus Selector3/1
  Bus Selector3/2 -> Mux4/2  "<Y_G>"
  Bus Selector3/3 -> Mux4/3  "<Z_G>"
  Track Data/1(gamma) -> Bus Creator7/1  "gamma"
  Track Data/2(Chi) -> Bus Creator7/2  "Chi"
  Bus Creator7/1 -> Bus Creator5/2  "TrackData"

== system AircraftModel_6DoF_SAS/Flight Controls ==
  Inp : Inport
  EoM : Inport  Port=2  OutDataTypeStr=Bus: EoM
  Aero : Inport  Port=3  OutDataTypeStr=Bus: Aero
  Bus Creator1 : BusCreator  Inputs=4  OutDataTypeStr=Bus: Cmd
  Lateral Directional Control Laws : Subsystem
  Longitudinal Control Laws1 : Subsystem
  Cmd : Outport  OutDataTypeStr=Bus: Cmd
  wires:
  Inp/1 -> Longitudinal Control Laws1/3(Inp), Lateral Directional Control Laws/3(Inp)
  Bus Creator1/1 -> Cmd/1  "Cmd"
  Lateral Directional Control Laws/2(cmd_dr) -> Bus Creator1/3  "cmd_dr"
  EoM/1 -> Longitudinal Control Laws1/2(EoM), Lateral Directional Control Laws/2(EoM)
  Longitudinal Control Laws1/1(cmd_de) -> Bus Creator1/1  "cmd_de"
  Lateral Directional Control Laws/1(cmd_da) -> Bus Creator1/2  "cmd_da"
  Longitudinal Control Laws1/2(cmd_dt) -> Bus Creator1/4  "cmd_dt"
  Aero/1 -> Longitudinal Control Laws1/1(Aero), Lateral Directional Control Laws/1(Aero)

== system AircraftModel_6DoF_SAS/Gravity ==
  note: Gravitational Force
  EoM : Inport  OutDataTypeStr=Bus: EoM
  Bus Creator : BusCreator  Inputs=3  OutDataTypeStr=Bus: Grav
  Bus Selector : BusSelector  OutputSignals=CC.CC_fg
  CC_fg * gg : Product  Multiplication=Matrix(*)  RndMeth=Zero
  Demux : Demux  Outputs=3
  Grav. Acc. : Constant  Value=CNT_g  SampleTime=-1
  Grav : Outport  OutDataTypeStr=Bus: Grav
  wires:
  EoM/1 -> Bus Selector/1
  Bus Selector/1 -> CC_fg * gg/1  "<CC_fg>"
  CC_fg * gg/1 -> Demux/1  "gg_f"
  Grav. Acc./1 -> CC_fg * gg/2  "gg"
  Demux/1 -> Bus Creator/1  "X_G"
  Demux/2 -> Bus Creator/2  "Y_G"
  Demux/3 -> Bus Creator/3  "Z_G"
  Bus Creator/1 -> Grav/1

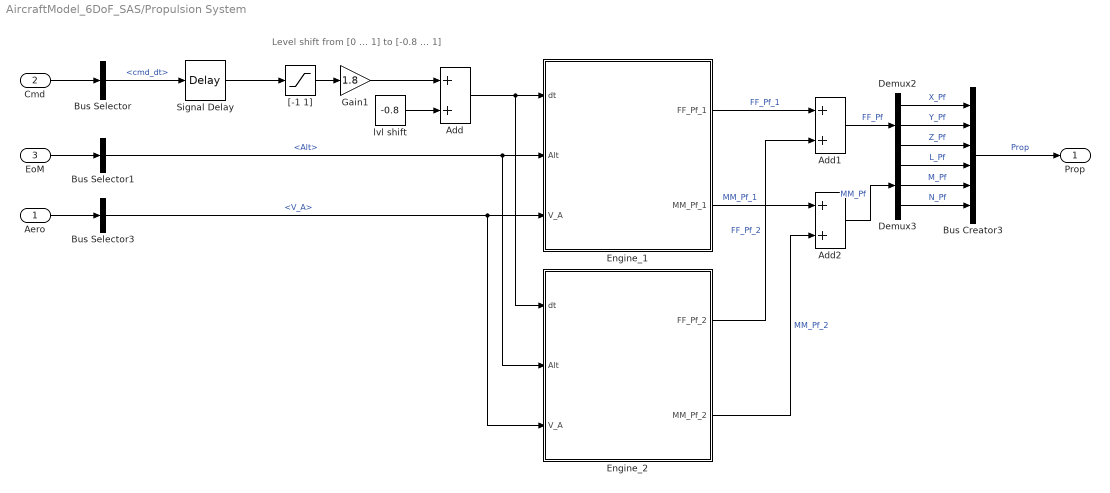
== system AircraftModel_6DoF_SAS/Propulsion System  ==
  note: Level shift from [0 ... 1] to [-0.8 ... 1]
  Aero : Inport  OutDataTypeStr=Bus: Aero
  Cmd : Inport  Port=2  OutDataTypeStr=Bus: Cmd
  EoM : Inport  Port=3  OutDataTypeStr=Bus: EoM
  Add : Sum
  Add1 : Sum
  Add2 : Sum
  Bus Creator3 : BusCreator  Inputs=6  OutDataTypeStr=Bus: Prop
  Bus Selector : BusSelector  OutputSignals=cmd_dt
  Bus Selector1 : BusSelector  OutputSignals=Position.Alt
  Bus Selector3 : BusSelector  OutputSignals=AirData.V_A
  Demux2 : Demux  Outputs=3
  Demux3 : Demux  Outputs=3
  Engine_1 : Subsystem
  Engine_2 : Subsystem
  Gain1 : Gain  Gain=1.8
  Signal Delay : TransportDelay  DelayTime=Propulsion.Delays.tau_dt  InitialOutput=TrimPoint.States.dtbar  TransDelayFeedthrough=on
  "[-1 1]" : Saturate  UpperLimit=1  LowerLimit=0
  lvl shift : Constant  Value=-0.8  SampleTime=-1
  Prop : Outport  OutDataTypeStr=Bus: Prop
  wires:
  Demux2/2 -> Bus Creator3/2  "Y_Pf"
  Engine_1/1(FF_Pf_1) -> Add1/1  "FF_Pf_1"
  Demux3/1 -> Bus Creator3/4  "L_Pf"
  EoM/1 -> Bus Selector1/1
  lvl shift/1 -> Add/2
  Engine_2/1(FF_Pf_2) -> Add1/2  "FF_Pf_2"
  Add2/1 -> Demux3/1  "MM_Pf"
  Bus Selector3/1 -> Engine_2/3(V_A), Engine_1/3(V_A)  "<V_A>"
  Aero/1 -> Bus Selector3/1
  Demux2/1 -> Bus Creator3/1  "X_Pf"
  Gain1/1 -> Add/1
  Engine_1/2(MM_Pf_1) -> Add2/1  "MM_Pf_1"
  Add/1 -> Engine_2/1(dt), Engine_1/1(dt)
  Bus Creator3/1 -> Prop/1  "Prop"
  Demux3/2 -> Bus Creator3/5  "M_Pf"
  "[-1 1]"/1 -> Gain1/1
  Demux2/3 -> Bus Creator3/3  "Z_Pf"
  Add1/1 -> Demux2/1  "FF_Pf"
  Bus Selector1/1 -> Engine_2/2(Alt), Engine_1/2(Alt)  "<Alt>"
  Demux3/3 -> Bus Creator3/6  "N_Pf"
  Cmd/1 -> Bus Selector/1
  Bus Selector/1 -> Signal Delay/1  "<cmd_dt>"
  Engine_2/2(MM_Pf_2) -> Add2/2  "MM_Pf_2"
  Signal Delay/1 -> "[-1 1]"/1

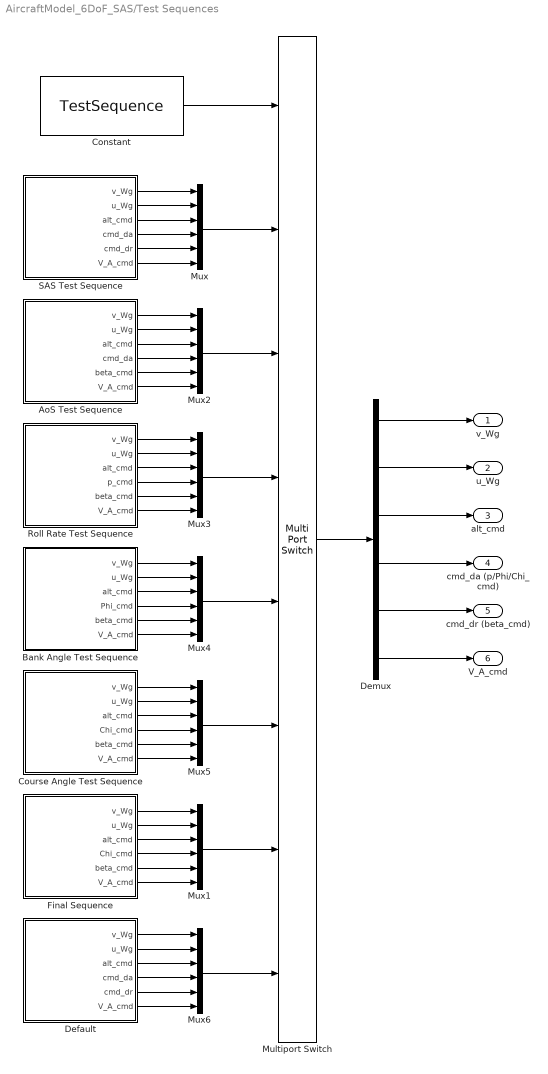
== system AircraftModel_6DoF_SAS/Test Sequences ==
  AoS Test Sequence : Subsystem
  Bank Angle Test Sequence : Subsystem
  Constant : Constant  Value=TestSequence
  Course Angle Test Sequence : Subsystem
  Default : Subsystem
  Demux : Demux  Outputs=6
  Final Sequence : Subsystem
  Multiport Switch : MultiPortSwitch  Inputs=7
  Mux{,1..6} (7 alike) : Mux  Inputs=6
  Roll Rate Test Sequence : Subsystem
  SAS Test Sequence : Subsystem
  v_Wg : Outport
  u_Wg : Outport  Port=2
  alt_cmd : Outport  Port=3
  cmd_da (p/Phi/Chi_cmd) : Outport  Port=4
  cmd_dr (beta_cmd) : Outport  Port=5
  V_A_cmd : Outport  Port=6
  wires:
  SAS Test Sequence/1(v_Wg) -> Mux/1
  SAS Test Sequence/2(u_Wg) -> Mux/2
  SAS Test Sequence/3(alt_cmd) -> Mux/3
  SAS Test Sequence/4(cmd_da) -> Mux/4
  SAS Test Sequence/5(cmd_dr) -> Mux/5
  SAS Test Sequence/6(V_A_cmd) -> Mux/6
  Final Sequence/1(v_Wg) -> Mux1/1
  Final Sequence/2(u_Wg) -> Mux1/2
  Final Sequence/3(alt_cmd) -> Mux1/3
  Final Sequence/4(Chi_cmd) -> Mux1/4
  Final Sequence/5(beta_cmd) -> Mux1/5
  Final Sequence/6(V_A_cmd) -> Mux1/6
  AoS Test Sequence/6(V_A_cmd) -> Mux2/6
  AoS Test Sequence/5(beta_cmd) -> Mux2/5
  AoS Test Sequence/4(cmd_da) -> Mux2/4
  AoS Test Sequence/3(alt_cmd) -> Mux2/3
  AoS Test Sequence/2(u_Wg) -> Mux2/2
  AoS Test Sequence/1(v_Wg) -> Mux2/1
  Roll Rate Test Sequence/1(v_Wg) -> Mux3/1
  Roll Rate Test Sequence/5(beta_cmd) -> Mux3/5
  Roll Rate Test Sequence/2(u_Wg) -> Mux3/2
  Roll Rate Test Sequence/4(p_cmd) -> Mux3/4
  Roll Rate Test Sequence/3(alt_cmd) -> Mux3/3
  Roll Rate Test Sequence/6(V_A_cmd) -> Mux3/6
  Bank Angle Test Sequence/1(v_Wg) -> Mux4/1
  Bank Angle Test Sequence/2(u_Wg) -> Mux4/2
  Bank Angle Test Sequence/3(alt_cmd) -> Mux4/3
  Bank Angle Test Sequence/4(Phi_cmd) -> Mux4/4
  Bank Angle Test Sequence/5(beta_cmd) -> Mux4/5
  Bank Angle Test Sequence/6(V_A_cmd) -> Mux4/6
  Course Angle Test Sequence/4(Chi_cmd) -> Mux5/4
  Course Angle Test Sequence/5(beta_cmd) -> Mux5/5
  Course Angle Test Sequence/2(u_Wg) -> Mux5/2
  Course Angle Test Sequence/1(v_Wg) -> Mux5/1
  Course Angle Test Sequence/3(alt_cmd) -> Mux5/3
  Course Angle Test Sequence/6(V_A_cmd) -> Mux5/6
  Multiport Switch/1 -> Demux/1
  Demux/1 -> v_Wg/1
  Demux/2 -> u_Wg/1
  Demux/3 -> alt_cmd/1
  Demux/4 -> cmd_da (p/Phi/Chi_cmd)/1
  Demux/5 -> cmd_dr (beta_cmd)/1
  Demux/6 -> V_A_cmd/1
  Mux/1 -> Multiport Switch/2
  Mux2/1 -> Multiport Switch/3
  Mux3/1 -> Multiport Switch/4
  Mux4/1 -> Multiport Switch/5
  Mux5/1 -> Multiport Switch/6
  Constant/1 -> Multiport Switch/1
  Default/6(V_A_cmd) -> Mux6/6
  Default/5(cmd_dr) -> Mux6/5
  Default/4(cmd_da) -> Mux6/4
  Default/3(alt_cmd) -> Mux6/3
  Default/2(u_Wg) -> Mux6/2
  Default/1(v_Wg) -> Mux6/1
  Mux1/1 -> Multiport Switch/7
  Mux6/1 -> Multiport Switch/8

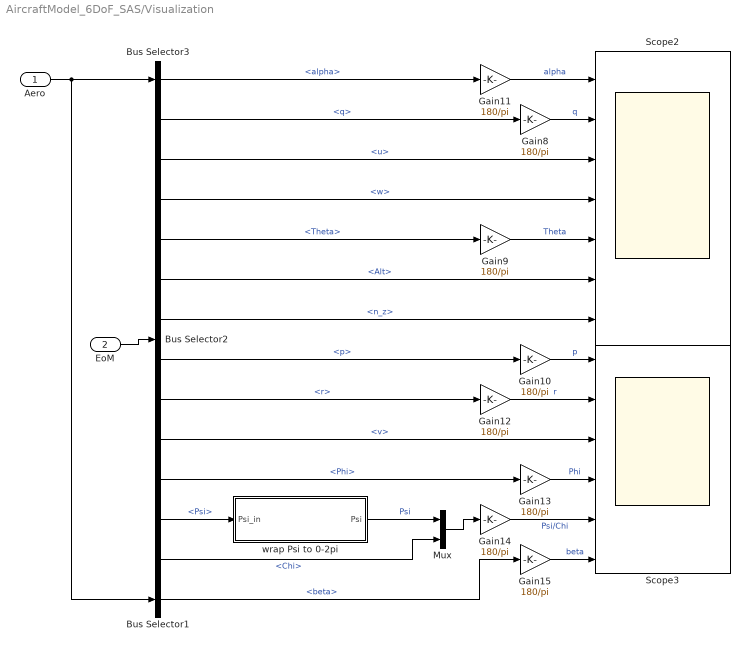
== system AircraftModel_6DoF_SAS/Visualization ==
  Aero : Inport  OutDataTypeStr=Bus: Aero
  EoM : Inport  Port=2  OutDataTypeStr=Bus: EoM
  Bus Selector1 : BusSelector  OutputSignals=AirData.beta
  Bus Selector2 : BusSelector  OutputSignals=OOmega_f.q,vv_f.u,vv_f.w,PPhi.Theta,Position.Alt,nn_f.n_z,OOmega_f.p,OOmega_f.r,vv_f.v,PPhi.Phi,PPhi.Psi,TrackData.Chi
  Bus Selector3 : BusSelector  OutputSignals=AirData.alpha
  Gain{8..15} (8 alike) : Gain  Gain=180/pi
  Mux : Mux  Inputs=2
  Scope2 : Scope  NumInputPorts=7
  Scope3 : Scope  NumInputPorts=6
  wrap Psi to 0-2pi : MATLAB Function  TreatAsAtomicUnit=on
  wires:
  Bus Selector2/8 -> Gain12/1  "<r>"
  Gain8/1 -> Scope2/2  "q"
  Gain13/1 -> Scope3/4  "Phi"
  Gain12/1 -> Scope3/2  "r"
  Gain15/1 -> Scope3/6  "beta"
  Gain11/1 -> Scope2/1  "alpha"
  Gain14/1 -> Scope3/5  "Psi/Chi"
  Gain9/1 -> Scope2/5  "Theta"
  Gain10/1 -> Scope3/1  "p"
  Aero/1 -> Bus Selector3/1, Bus Selector1/1
  Bus Selector2/9 -> Scope3/3  "<v>"
  Bus Selector2/2 -> Scope2/3  "<u>"
  Bus Selector2/1 -> Gain8/1  "<q>"
  EoM/1 -> Bus Selector2/1
  Bus Selector2/6 -> Scope2/7  "<n_z>"
  Bus Selector2/11 -> wrap Psi to 0-2pi/1(Psi_in)  "<Psi>"
  Bus Selector2/5 -> Scope2/6  "<Alt>"
  Bus Selector3/1 -> Gain11/1  "<alpha>"
  Bus Selector2/10 -> Gain13/1  "<Phi>"
  Bus Selector2/3 -> Scope2/4  "<w>"
  Bus Selector2/7 -> Gain10/1  "<p>"
  Bus Selector2/4 -> Gain9/1  "<Theta>"
  Bus Selector1/1 -> Gain15/1  "<beta>"
  Bus Selector2/12 -> Mux/2  "<Chi>"
  Mux/1 -> Gain14/1
  wrap Psi to 0-2pi/1(Psi) -> Mux/1  "Psi"

== system AircraftModel_6DoF_SAS/Equations of Motion/Calculation of Position_dot ==
  Position : Inport  OutDataTypeStr=Bus: Position
  vv_g : Inport  Port=2
  " " : Trigonometry  Operator=cos
  Alt_dot : Gain  Gain=-1
  Bus Selector2 : BusSelector  OutputSignals=Alt,Lat
  CNT_a : Constant  Value=CNT_a  SampleTime=-1
  CNT_f : Constant  Value=CNT_f  SampleTime=-1
  Demux : Demux  Outputs=3
  Lat_dot : Product  Inputs=*/
  Lon_dot : Product  Inputs=/*/
  Mux : Mux  Inputs=3
  Sum : Sum  Inputs=++|
  Sum1 : Sum  Inputs=++|
  WGS84 : MATLAB Function  TreatAsAtomicUnit=on
  ZeroOffset - cos (Lat) : Subsystem  mask(Zero offset){tol=1E-5}
      mask prompts: tol "Tolerance"
      mask help: This block outputs a value equal to the tolerance specified in the block parameters if the input falls within a sphere with this tolerance as radius and center in the origin. Otherwise, the output equals the input.
      mask Help: This block outputs a value equal to the tolerance specified in the block parameters if the input falls within a sphere with this tolerance as radius and center in the origin. Otherwise, the output equals the input.
  Position_dot : Outport
  wires:
  ZeroOffset - cos (Lat)/1(Out) -> Lon_dot/3
  Mux/1 -> Position_dot/1  "Position_dot"
  vv_g/1 -> Demux/1  "vv_g"
  Position/1 -> Bus Selector2/1  "Position"
  Lat_dot/1 -> Mux/1  "Lat_dot"
  Lon_dot/1 -> Mux/2  "Lon_dot"
  Alt_dot/1 -> Mux/3  "Alt_dot"
  Demux/3 -> Alt_dot/1  "w_g"
  Demux/1 -> Lat_dot/1  "u_g"
  Demux/2 -> Lon_dot/2  "v_g"
  Sum/1 -> Lon_dot/1
  Sum1/1 -> Lat_dot/2
  WGS84/2(R_N) -> Sum/1
  WGS84/1(R_M) -> Sum1/1
  Bus Selector2/1 -> Sum1/2, Sum/2  "<Alt>"
  " "/1 -> ZeroOffset - cos (Lat)/1(In)
  Bus Selector2/2 -> WGS84/3(Lat), " "/1  "<Lat>"
  CNT_a/1 -> WGS84/1(CNT_a)  "CNT_a"
  CNT_f/1 -> WGS84/2(CNT_f)  "CNT_f"

== system AircraftModel_6DoF_SAS/Equations of Motion/INT_OOmega_f ==
  OOmega_dot_f : Inport
  Demux : Demux  Outputs=3
  INT_p : Integrator  InitialCondition=TrimPoint.States.pbar  ContinuousStateAttributes='p'
  INT_q : Integrator  InitialCondition=TrimPoint.States.qbar  ContinuousStateAttributes='q'
  INT_r : Integrator  InitialCondition=TrimPoint.States.rbar  ContinuousStateAttributes='r'
  Mux : Mux  Inputs=3
  Saturation : Saturate  UpperLimit=100000  LowerLimit=-100000
  Saturation1 : Saturate  UpperLimit=100000  LowerLimit=-100000
  Saturation2 : Saturate  UpperLimit=100000  LowerLimit=-100000
  OOmega_f : Outport
  wires:
  Mux/1 -> OOmega_f/1  "OOmega_f"
  INT_r/1 -> Mux/3  "r"
  INT_q/1 -> Mux/2  "q"
  INT_p/1 -> Mux/1  "p"
  Demux/3 -> Saturation2/1  "r_dot"
  Demux/2 -> Saturation1/1  "q_dot"
  Demux/1 -> Saturation/1  "p_dot"
  OOmega_dot_f/1 -> Demux/1  "OOmega_dot_f"
  Saturation/1 -> INT_p/1
  Saturation1/1 -> INT_q/1
  Saturation2/1 -> INT_r/1

== system AircraftModel_6DoF_SAS/Equations of Motion/INT_PPhi ==
  PPhi_dot : Inport
  Demux : Demux  Outputs=3
  INT_Phi : Integrator  InitialCondition=TrimPoint.States.Phibar  ContinuousStateAttributes='Phi'
  INT_Psi : Integrator  InitialCondition=TrimPoint.States.Psibar  ContinuousStateAttributes='Psi'
  INT_Theta : Integrator  InitialCondition=TrimPoint.States.Thetabar  ContinuousStateAttributes='Theta'
  Mux : Mux  Inputs=3
  Saturation : Saturate  UpperLimit=100000  LowerLimit=-100000
  Saturation1 : Saturate  UpperLimit=100000  LowerLimit=-100000
  Saturation2 : Saturate  UpperLimit=100000  LowerLimit=-100000
  PPhi : Outport
  wires:
  Saturation2/1 -> INT_Psi/1
  Saturation1/1 -> INT_Theta/1
  Saturation/1 -> INT_Phi/1
  Mux/1 -> PPhi/1  "PPhi"
  INT_Psi/1 -> Mux/3  "Psi"
  INT_Theta/1 -> Mux/2  "Theta"
  INT_Phi/1 -> Mux/1  "Phi"
  Demux/3 -> Saturation2/1  "Psi_dot"
  Demux/2 -> Saturation1/1  "Theta_dot"
  Demux/1 -> Saturation/1  "Phi_dot"
  PPhi_dot/1 -> Demux/1  "PPhi_dot"

== system AircraftModel_6DoF_SAS/Equations of Motion/INT_Position ==
  Position_dot : Inport
  Demux : Demux  Outputs=3
  INT_Alt : Integrator  InitialCondition=TrimPoint.States.Altbar  ContinuousStateAttributes='Alt'
  INT_Lat : Integrator  InitialCondition=TrimPoint.States.Latbar  ContinuousStateAttributes='Lat'
  INT_Lon : Integrator  InitialCondition=TrimPoint.States.Lonbar  ContinuousStateAttributes='Lon'
  Mux : Mux  Inputs=3
  Saturation : Saturate  UpperLimit=100000  LowerLimit=-100000
  Saturation1 : Saturate  UpperLimit=100000  LowerLimit=-100000
  Saturation2 : Saturate  UpperLimit=100000  LowerLimit=-100000
  Position : Outport
  wires:
  Saturation2/1 -> INT_Alt/1
  Saturation1/1 -> INT_Lon/1
  Saturation/1 -> INT_Lat/1
  Position_dot/1 -> Demux/1  "Position_dot"
  Demux/1 -> Saturation/1
  Demux/2 -> Saturation1/1
  Demux/3 -> Saturation2/1
  INT_Lat/1 -> Mux/1  "Lat"
  INT_Lon/1 -> Mux/2  "Lon"
  INT_Alt/1 -> Mux/3  "Alt"
  Mux/1 -> Position/1  "Position"

== system AircraftModel_6DoF_SAS/Equations of Motion/INT_vv_f ==
  vv_dot_f : Inport
  Demux : Demux  Outputs=3
  INT_u : Integrator  InitialCondition=TrimPoint.States.ubar  ContinuousStateAttributes='u'
  INT_v : Integrator  InitialCondition=TrimPoint.States.vbar  ContinuousStateAttributes='v'
  INT_w : Integrator  InitialCondition=TrimPoint.States.wbar  ContinuousStateAttributes='w'
  Mux : Mux  Inputs=3
  Saturation : Saturate  UpperLimit=100000  LowerLimit=-100000
  Saturation1 : Saturate  UpperLimit=100000  LowerLimit=-100000
  Saturation2 : Saturate  UpperLimit=100000  LowerLimit=-100000
  vv_f : Outport
  wires:
  vv_dot_f/1 -> Demux/1  "vv_dot_f"
  Demux/1 -> Saturation/1  "u_dot"
  Demux/2 -> Saturation1/1  "v_dot"
  Demux/3 -> Saturation2/1  "w_dot"
  INT_u/1 -> Mux/1  "u"
  INT_v/1 -> Mux/2  "v"
  INT_w/1 -> Mux/3  "w"
  Mux/1 -> vv_f/1  "vv_f"
  Saturation/1 -> INT_u/1
  Saturation1/1 -> INT_v/1
  Saturation2/1 -> INT_w/1

== system AircraftModel_6DoF_SAS/Equations of Motion/Latitude Bound ==
  In : Inport
  2pi : Constant  Value=2*pi  SampleTime=-1
  ChSign : Gain  Gain=-1  SaturateOnIntegerOverflow=on  OutDataTypeStr=Inherit: Same as input  ParamDataTypeStr=Inherit: Same as input
  Math Function : Math  Operator=mod  SignedPower=on  SaturateOnIntegerOverflow=on
  Math Function1 : Math  Operator=mod  SignedPower=on  SaturateOnIntegerOverflow=on
  Sum1 : Sum  Inputs=|+-  InputSameDT=on  SaturateOnIntegerOverflow=on  OutDataTypeStr=Inherit: Same as first input
  Sum2 : Sum  Inputs=|++  InputSameDT=on  SaturateOnIntegerOverflow=on  OutDataTypeStr=Inherit: Same as first input
  Switch : Switch  Threshold=pi  SaturateOnIntegerOverflow=on  InputSameDT=on
  pi : Constant  Value=pi  SampleTime=-1
  pi/2 : Constant  Value=pi/2  SampleTime=-1
  Out : Outport
  wires:
  pi/1 -> Math Function/2
  Math Function/1 -> Sum1/1
  pi/2/1 -> Sum1/2, Sum2/2
  Sum1/1 -> ChSign/1, Switch/3
  Math Function1/1 -> Switch/2
  Switch/1 -> Out/1
  In/1 -> Sum2/1
  Sum2/1 -> Math Function/1, Math Function1/1
  ChSign/1 -> Switch/1
  2pi/1 -> Math Function1/2

== system AircraftModel_6DoF_SAS/Equations of Motion/Longitude Bound ==
  In : Inport
  2pi : Constant  Value=2*pi  SampleTime=-1
  Math Function : Math  Operator=mod  SignedPower=on  SaturateOnIntegerOverflow=on
  Sum1 : Sum  Inputs=|+-  InputSameDT=on  SaturateOnIntegerOverflow=on  OutDataTypeStr=Inherit: Same as first input
  Sum2 : Sum  Inputs=|++  InputSameDT=on  SaturateOnIntegerOverflow=on  OutDataTypeStr=Inherit: Same as first input
  pi : Constant  Value=pi  SampleTime=-1
  Out : Outport
  wires:
  Sum1/1 -> Out/1
  pi/1 -> Sum1/2, Sum2/2
  Sum2/1 -> Math Function/1
  In/1 -> Sum2/1
  2pi/1 -> Math Function/2
  Math Function/1 -> Sum1/1

== system AircraftModel_6DoF_SAS/Equations of Motion/Track Data ==
  vv_g : Inport
  PPhi : Inport  Port=2  OutDataTypeStr=Bus: PPhi
  Alt_dot : Gain  Gain=-1
  Bus Selector : BusSelector  OutputSignals=Psi
  Chi1 : MATLAB Function  TreatAsAtomicUnit=on
  Demux : Demux  Outputs=3
  Product : Product  Inputs=/*
  Sin : Trigonometry  Operator=atan
  Terminator : Terminator
  gamma : Outport
  Chi : Outport  Port=2
  wires:
  Sin/1 -> gamma/1  "gamma"
  Demux/1 -> Product/1  "u_g"
  Product/1 -> Sin/1
  Demux/3 -> Alt_dot/1  "w_g"
  Alt_dot/1 -> Product/2  "Alt_dot"
  vv_g/1 -> Chi1/1(vv_g), Demux/1  "vv_g"
  Chi1/1(Chi) -> Chi/1  "Chi"
  Demux/2 -> Terminator/1  "v_g"
  PPhi/1 -> Bus Selector/1  "PPhi"
  Bus Selector/1 -> Chi1/2(Psi)  "<Psi>"

== system AircraftModel_6DoF_SAS/Flight Controls/Lateral Directional Control Laws ==
  Aero : Inport  OutDataTypeStr=Bus: Aero
  EoM : Inport  Port=2  OutDataTypeStr=Bus: EoM
  Inp : Inport  Port=3
  Demux : Demux  Outputs=2
  Saturation : Saturate  UpperLimit=max(Actuators.Limits.u_max_Hr)  LowerLimit=min(Actuators.Limits.u_max_Hr)
  Saturation1 : Saturate  UpperLimit=max(Actuators.Limits.u_max_Ha)  LowerLimit=min(Actuators.Limits.u_max_Ha)
  Selector : Selector  InputPortWidth=4  IndexOptions=Index vector (dialog)  Indices=[2 3]  OutputSizes=1
  Terminator1 : Terminator
  Terminator3 : Terminator
  cmd_da : Outport
  cmd_dr : Outport  Port=2
  wires:
  EoM/1 -> Terminator3/1
  Inp/1 -> Selector/1  "Inp"
  Aero/1 -> Terminator1/1
  Demux/1 -> Saturation1/1
  Selector/1 -> Demux/1
  Saturation1/1 -> cmd_da/1  "cmd_da"
  Demux/2 -> Saturation/1
  Saturation/1 -> cmd_dr/1  "cmd_dr"

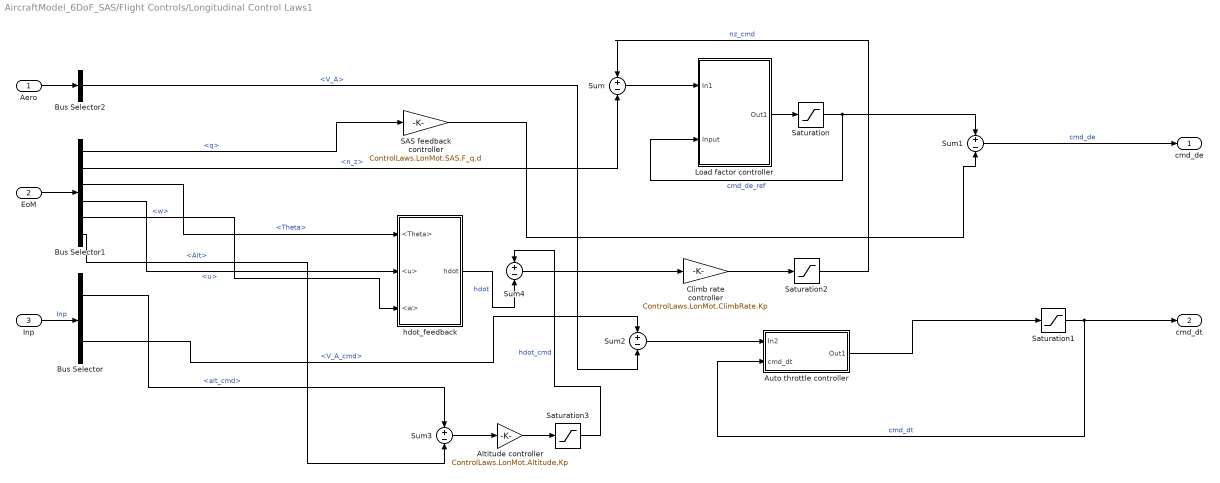
== system AircraftModel_6DoF_SAS/Flight Controls/Longitudinal Control Laws1 ==
  Aero : Inport  OutDataTypeStr=Bus: Aero
  EoM : Inport  Port=2  OutDataTypeStr=Bus: EoM
  Inp : Inport  Port=3
  Altitude controller : Gain  Gain=ControlLaws.LonMot.Altitude.Kp
  Auto throttle controller : Subsystem
  Bus Selector : BusSelector  OutputSignals=alt_cmd,V_A_cmd
  Bus Selector1 : BusSelector  OutputSignals=OOmega_f.q,nn_f.n_z,PPhi.Theta,vv_f.u,vv_f.w,Position.Alt
  Bus Selector2 : BusSelector  OutputSignals=AirData.V_A
  Climb rate controller : Gain  Gain=ControlLaws.LonMot.ClimbRate.Kp
  Load factor controller : Subsystem
  SAS feedback controller : Gain  Gain=ControlLaws.LonMot.SAS.F_q.d
  Saturation : Saturate  UpperLimit=Actuators.Limits.u_max_He(2)  LowerLimit=Actuators.Limits.u_max_He(1)
  Saturation1 : Saturate  UpperLimit=1  LowerLimit=0
  Saturation2 : Saturate  UpperLimit=ControlLaws.Saturations.nz(2)  LowerLimit=ControlLaws.Saturations.nz(1)  LinearizeAsGain=off
  Saturation3 : Saturate  UpperLimit=ControlLaws.Saturations.hdot(2)  LowerLimit=ControlLaws.Saturations.hdot(1)
  Sum{,1..4} (5 alike) : Sum  Inputs=+-
  hdot_feedback : Subsystem
  cmd_de : Outport
  cmd_dt : Outport  Port=2
  wires:
  Inp/1 -> Bus Selector/1  "Inp"
  EoM/1 -> Bus Selector1/1
  Bus Selector1/1 -> SAS feedback controller/1  "<q>"
  Aero/1 -> Bus Selector2/1
  Bus Selector1/2 -> Sum/2  "<n_z>"
  Sum/1 -> Load factor controller/1(In1)
  Load factor controller/1(Out1) -> Saturation/1
  Saturation/1 -> Sum1/1, Load factor controller/2(Input)  "cmd_de_ref"
  SAS feedback controller/1 -> Sum1/2
  Sum1/1 -> cmd_de/1  "cmd_de"
  Saturation1/1 -> cmd_dt/1, Auto throttle controller/2(cmd_dt)  "cmd_dt"
  Bus Selector2/1 -> Sum2/2  "<V_A>"
  Sum2/1 -> Auto throttle controller/1(In2)
  Auto throttle controller/1(Out1) -> Saturation1/1
  Bus Selector1/3 -> hdot_feedback/1(<Theta>)  "<Theta>"
  Bus Selector1/4 -> hdot_feedback/2(<u>)  "<u>"
  Bus Selector1/5 -> hdot_feedback/3(<w>)  "<w>"
  Climb rate controller/1 -> Saturation2/1
  Bus Selector1/6 -> Sum3/2  "<Alt>"
  Sum3/1 -> Altitude controller/1
  Altitude controller/1 -> Saturation3/1
  hdot_feedback/1(hdot) -> Sum4/2  "hdot"
  Bus Selector/2 -> Sum2/1  "<V_A_cmd>"
  Sum4/1 -> Climb rate controller/1
  Saturation2/1 -> Sum/1  "nz_cmd"
  Bus Selector/1 -> Sum3/1  "<alt_cmd>"
  Saturation3/1 -> Sum4/1  "hdot_cmd"
